simulink model "Systolic_Associative_4_tap"  (R2021a)
settings: Solver=VariableStepAuto  StartTime=0.0  StopTime=4000  RelTol=1e-3
undefined symbols (not defined in the file): variable_step_size_calc, variable_step_size_calc_1, x1
libraries: dspsrcs4 x4, dspstat3 x4, dspmathops x2
settings Model: Creator=HP  LastModifiedBy=HP

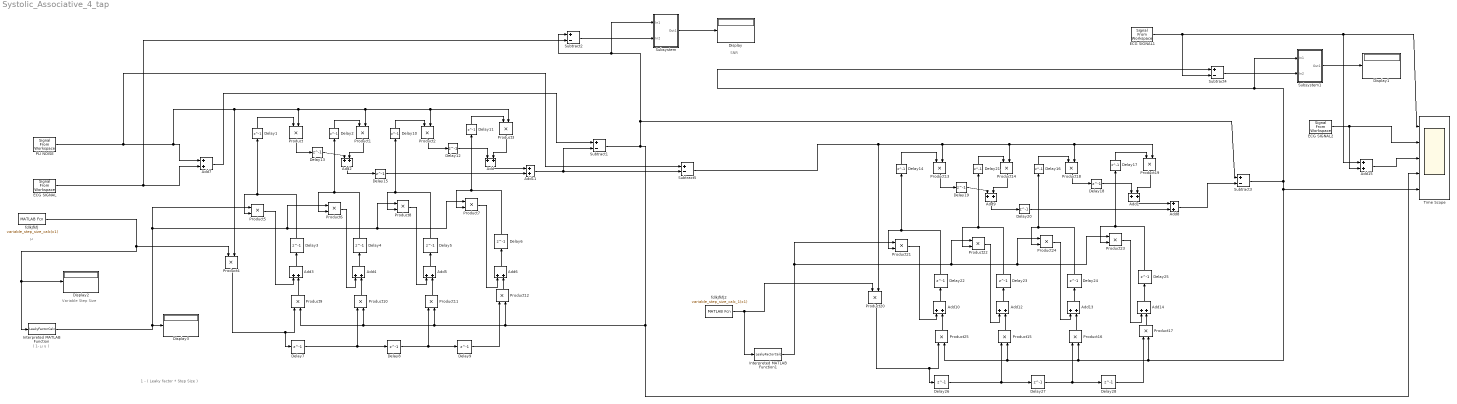
== system Systolic_Associative_4_tap ==
  note: SNR
  note: μ
  note: Variable Step Size
  note: 1 - ( Leaky factor * Step Size )
  note: ( 1- μ γ )
  Add{,1..15} (16 alike) : Sum
  Delay{1..28} (28 alike) : Delay  DelayLength=1  InitialCondition=0
  Display{,1..3} (4 alike) : Display
      Display3 settings: Format=decimal (Stored Integer)
  ECG SIGNAL : dspsrcs4/Signal From Workspace  X=m1  Ts=1  nsamps=1  OutputAfterFinalValue=Setting to zero  ignoreOrWarnInputAndFrameLengths=off  OutputFrames=off
  ECG SIGNAL1 : dspsrcs4/Signal From Workspace  X=m1  Ts=1  nsamps=1  OutputAfterFinalValue=Setting to zero  ignoreOrWarnInputAndFrameLengths=off  OutputFrames=off
  ECG SIGNAL2 : dspsrcs4/Signal From Workspace  X=x1  Ts=1  nsamps=1  OutputAfterFinalValue=Setting to zero  ignoreOrWarnInputAndFrameLengths=off  OutputFrames=off
  Interpreted MATLAB Function : MATLABFcn  MATLABFcn=LeakyFactorCalc
  Interpreted MATLAB Function1 : MATLABFcn  MATLABFcn=LeakyFactorCalc
  PLI NOISE : dspsrcs4/Signal From Workspace  X=x1  Ts=1  nsamps=1  OutputAfterFinalValue=Setting to zero  ignoreOrWarnInputAndFrameLengths=off  OutputFrames=off
  Product{,1..25} (26 alike) : Product
  Subsystem : Subsystem
  Subsystem1 : Subsystem
  Subtract{1..5} (5 alike) : Sum  Inputs=+-
  Time Scope : Scope  NumInputPorts=5
  fdlkjfkfj : MATLABFcn  MATLABFcn=variable_step_size_calc(x1)
  fdlkjfkfj2 : MATLABFcn  MATLABFcn=variable_step_size_calc_1(x1)
  wires:
  Delay2/1 -> Product1/1
  Delay1/1 -> Product/1
  Delay10/1 -> Product2/1
  Delay11/1 -> Product3/1
  Product6/1 -> Add4/1
  Delay5/1 -> Product8/2, Delay10/1
  Delay3/1 -> Delay1/1, Product5/2
  Product7/1 -> Add6/1
  Product5/1 -> Add3/1
  Product11/1 -> Add5/2
  Delay6/1 -> Product7/2, Delay11/1
  PLI NOISE/1 -> Subtract5/1, Add7/1, Product3/2, Product2/2, Product1/2, Product/2, Product4/2
  Delay8/1 -> Product11/1, Delay9/1
  Delay4/1 -> Delay2/1, Product6/2
  Add4/1 -> Delay4/1
  Product9/1 -> Add3/2
  Add7/1 -> Subtract1/1
  Delay9/1 -> Product12/1
  Add3/1 -> Delay3/1
  Add5/1 -> Delay5/1
  Delay7/1 -> Product10/1, Delay8/1
  Subtract2/1 -> Subsystem/2(In2)
  fdlkjfkfj/1 -> Product4/1, Interpreted MATLAB Function/1, Display2/1
  Product8/1 -> Add5/1
  Add6/1 -> Delay6/1
  ECG SIGNAL/1 -> Add7/2, Subtract2/2
  Product10/1 -> Add4/2
  Subsystem/1(Out1) -> Display/1
  Product12/1 -> Add6/2
  Product4/1 -> Product9/1, Delay7/1
  Product3/1 -> Add/2
  Product2/1 -> Delay12/1
  Delay12/1 -> Add/1
  Product/1 -> Delay13/1
  Delay13/1 -> Add2/1
  Product1/1 -> Add2/2
  Add2/1 -> Delay15/1
  Delay15/1 -> Add11/2
  Add/1 -> Add11/1
  Add11/1 -> Subtract5/2, Subtract1/2
  Add1/1 -> Add8/1
  Delay19/1 -> Add9/1
  Delay22/1 -> Delay14/1, Product21/2
  Product22/1 -> Add12/1
  Add8/1 -> Subtract3/2
  Add9/1 -> Delay20/1
  Product13/1 -> Delay19/1
  Product19/1 -> Add1/2
  Product15/1 -> Add12/2
  Product18/1 -> Delay18/1
  Delay27/1 -> Product16/1, Delay28/1
  Delay20/1 -> Add8/2
  Delay18/1 -> Add1/1
  Product17/1 -> Add14/2
  Add14/1 -> Delay25/1
  Subsystem1/1(Out1) -> Display1/1
  Product20/1 -> Product25/1, Delay26/1
  Product24/1 -> Add13/1
  Interpreted MATLAB Function/1 -> Display3/1, Product5/1, Product6/1, Product8/1, Product7/1
  Subtract5/1 -> Product19/2, Product18/2, Product14/2, Product13/2, Product20/2
  Product25/1 -> Add10/2
  Product23/1 -> Add14/1
  Product21/1 -> Add10/1
  Delay25/1 -> Product23/2, Delay17/1
  Delay21/1 -> Product14/1
  Add13/1 -> Delay24/1
  Product14/1 -> Add9/2
  Add12/1 -> Delay23/1
  Add10/1 -> Delay22/1
  Delay24/1 -> Product24/2, Delay16/1
  Subtract4/1 -> Subsystem1/2(In2)
  Delay26/1 -> Product15/1, Delay27/1
  Delay14/1 -> Product13/1
  Subtract3/1 -> Product17/2, Product16/2, Product15/2, Product25/2, Time Scope/5, Subsystem1/1(In1), Subtract4/1
  Product16/1 -> Add13/2
  Delay17/1 -> Product19/1
  Delay28/1 -> Product17/1
  Delay23/1 -> Delay21/1, Product22/2
  Delay16/1 -> Product18/1
  ECG SIGNAL1/1 -> Add15/1, Time Scope/1, Subtract4/2
  ECG SIGNAL2/1 -> Add15/2, Time Scope/2
  Add15/1 -> Time Scope/3
  Subtract1/1 -> Subtract3/1, Subsystem/1(In1), Subtract2/1, Time Scope/4, Product12/2, Product11/2, Product10/2, Product9/2
  fdlkjfkfj2/1 -> Interpreted MATLAB Function1/1, Product20/1
  Interpreted MATLAB Function1/1 -> Product24/1, Product23/1, Product22/1, Product21/1

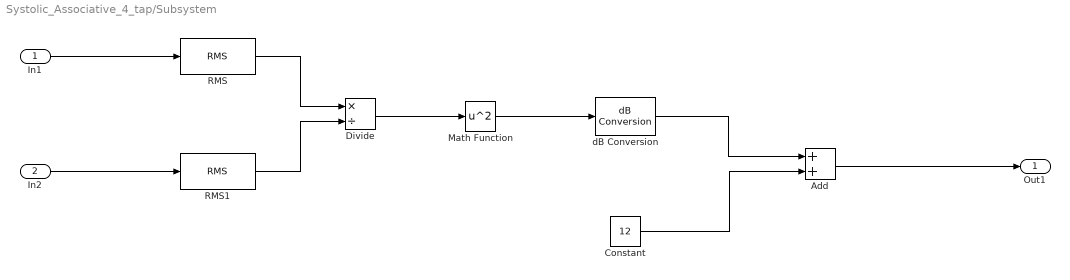
== system Systolic_Associative_4_tap/Subsystem ==
  In1 : Inport
  In2 : Inport  Port=2
  Add : Sum
  Constant : Constant  Value=12
  Divide : Product  Inputs=*/
  Math Function : Math  Operator=square  SignedPower=on  OutputSignalType=real  SaturateOnIntegerOverflow=on
  RMS : dspstat3/RMS  run=on  directionMode=Each column  dimension=1  InputProcessing=Columns as channels (frame based)  reset_popup=None
  RMS1 : dspstat3/RMS  run=on  directionMode=Each column  dimension=1  InputProcessing=Columns as channels (frame based)  reset_popup=None
  dB Conversion : dspmathops/dB Conversion  dBtype=dB  intype=Amplitude  R=1  fuzz=off
  Out1 : Outport
  wires:
  RMS1/1 -> Divide/2
  dB Conversion/1 -> Add/1
  In1/1 -> RMS/1
  Divide/1 -> Math Function/1
  RMS/1 -> Divide/1
  In2/1 -> RMS1/1
  Add/1 -> Out1/1
  Constant/1 -> Add/2
  Math Function/1 -> dB Conversion/1

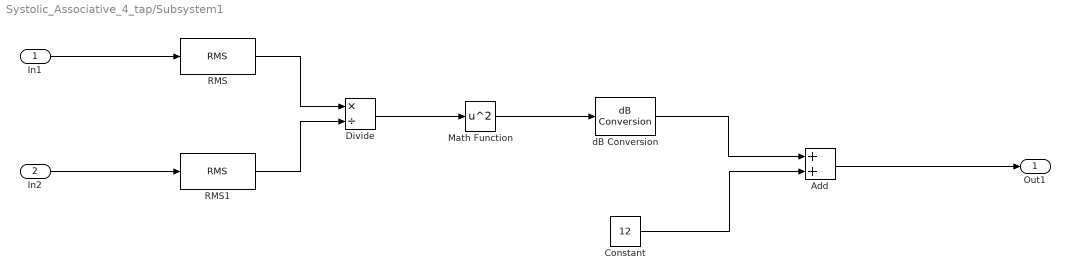
== system Systolic_Associative_4_tap/Subsystem1 ==
  In1 : Inport
  In2 : Inport  Port=2
  Add : Sum
  Constant : Constant  Value=12
  Divide : Product  Inputs=*/
  Math Function : Math  Operator=square  SignedPower=on  OutputSignalType=real  SaturateOnIntegerOverflow=on
  RMS : dspstat3/RMS  run=on  directionMode=Each column  dimension=1  InputProcessing=Columns as channels (frame based)  reset_popup=None
  RMS1 : dspstat3/RMS  run=on  directionMode=Each column  dimension=1  InputProcessing=Columns as channels (frame based)  reset_popup=None
  dB Conversion : dspmathops/dB Conversion  dBtype=dB  intype=Amplitude  R=1  fuzz=off
  Out1 : Outport
  wires:
  RMS1/1 -> Divide/2
  dB Conversion/1 -> Add/1
  In1/1 -> RMS/1
  Divide/1 -> Math Function/1
  RMS/1 -> Divide/1
  In2/1 -> RMS1/1
  Add/1 -> Out1/1
  Constant/1 -> Add/2
  Math Function/1 -> dB Conversion/1
